simulink model "Parallel_Servo"  (R2022b)
settings: Solver=FixedStepAuto  StartTime=0.0  StopTime=10  FixedStep=1e-3  RelTol=1e-3  EnableMultiTasking=on
undefined symbols (not defined in the file or in its folder): LF
libraries: instrumentseriallib x2
settings Model: ExtModeTrigDuration=2  Creator=gotta  LastModifiedBy=gotta
settings SolverCC: AutoInsertRateTranBlk=on
settings DataIOCC: SaveFormat=Array  SaveOutput=off  DSMLogging=off  SaveTime=off  ReturnWorkspaceOutputs=off
settings OptimizationCC: EnhancedBackFolding=on  PassReuseOutputArgsAs=Individual arguments  ZeroExternalMemoryAtStartup=off  ZeroInternalMemoryAtStartup=off  MaxStackSize=64  OptimizeBlockOrder=speed  DifferentSizesBufferReuse=on  OptimizationCustomize=off  EfficientTunableParamExpr=on
settings DebuggingCC: ParameterTunabilityLossMsg=error
settings HardwareCC: ProdBitPerInt=16  ProdBitPerPointer=16  ProdBitPerSizeT=16  ProdBitPerPtrDiffT=16  ProdLargestAtomicFloat=None  ProdWordSize=8  ProdHWDeviceType=Atmel->AVR
settings SFSimCC: MATLABDynamicMemAlloc=off
settings RTWCC: Description=Embedded Coder  SystemTargetFile=ert.tlc  HardwareBoard=Arduino Mega 2560  TLCOptions="-aInlineSetEventsForThisBaseRateFcn=TLC_FALSE -aSuppressMultiTaskScheduler=TLC_FALSE   -aRateBasedStepFcn=1"  TemplateMakefile=ert_default_tmf  Toolchain=Arduino AVR  BuildConfiguration=Faster Runs
settings CodeAppCC: ForceParamTrailComments=on  IgnoreCustomStorageClasses=off  OperatorAnnotations=on  SimulinkDataObjDesc=on  SFDataObjDesc=on  InsertBlockDesc=on
settings ERTTargetCC: TargetLangStandard=C99 (ISO)  SupportContinuousTime=on  SupportVariableSizeSignals=on  ExtModeTransport=3  ExtModeStaticAlloc=on  ExtModeAutomaticAllocSize=off  ExtModeStaticAllocSize=2048  ExtModeMexFile=ext_xcp  ExtModeIntrfLevel=Level2 - Open

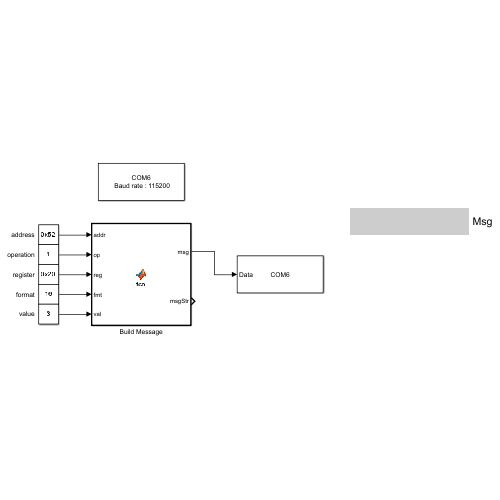
[thumbnail: Simulink's stored preview of the top-level diagram]
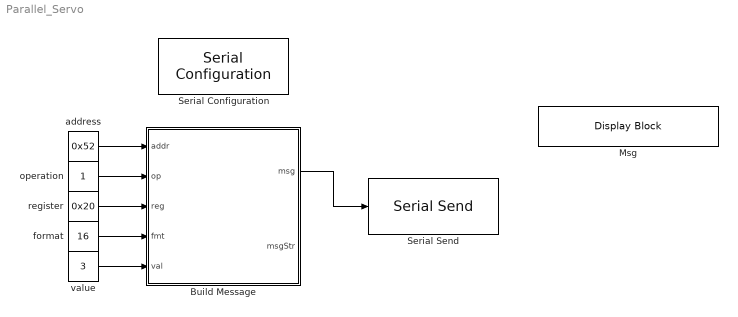
== system Parallel_Servo ==
  Build Message : MATLAB Function  TreatAsAtomicUnit=on
  Msg : DisplayBlock  LabelPosition=Hide  Transparency=1
  Serial Configuration : instrumentseriallib/Serial Configuration  Priority=-200000  PortSel=COM6  Port=COM6  ComPort=COM6  BaudRate=115200  DataBits=8  Parity=none  StopBits=1  ByteOrder=little-endian  FlowControl=none  Timeout=10  SimulateUsing=Interpreted execution  BlockInModel=on  aMode=1
  Serial Send : instrumentseriallib/Serial Send  Priority=1  PortSel=COM6  Port=COM6  ComPort=COM6  Header='A'  Terminator=LF ('\n')  CustomTerminator=[]  EnableBlockingMode=on  SimulateUsing=Interpreted execution  BlockInModel=on  aMode=1
  address : Constant  Value=0x52
  format : Constant  Value=16
  operation : Constant  OutDataTypeStr=boolean
  register : Constant  Value=0x20
  value : Constant  Value=3
  wires:
  Build Message/1(msg) -> Serial Send/1
  address/1 -> Build Message/1(addr)
  value/1 -> Build Message/5(val)
  format/1 -> Build Message/4(fmt)
  register/1 -> Build Message/3(reg)
  operation/1 -> Build Message/2(op)

== matlab function Parallel_Servo/Build Message ==
  data: addr input; msg output size=[1 32]; op input; reg input; fmt input; val input; msgStr output
function [msg, msgStr] = fcn(addr, op, reg, fmt, val)

% indirizzo
addr = toHexString(addr);

% operazione
if op
    op = "w";
else
    op = "r";
end

% registro
reg = toHexString(reg);

% formato
if fmt > 100
    tempFmt = 'i';
    fmt = fmt - 100;
else
    tempFmt = 'u';
end

fmt = tempFmt + string(fmt);

% messaggio
msg = zeros(1, 32, 'uint8');

msgStr = addr + " " + op + " " + reg + " " + fmt + " " + val;
msgBytes = uint8(char(msgStr));

msg(1:min(length(msgBytes), 32)) = msgBytes(1:min(length(msgBytes), 32));
msgStr = string(char(msg));

end
